simulink model "Messages4_2018a"  (R2018a)
settings: Solver=VariableStepAuto  StartTime=0.0  StopTime=0.2  RelTol=1e-3
settings Model: Creator=86188  LastModifiedBy=86188

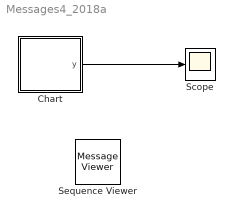
== system Messages4_2018a ==
  Chart : Stateflow chart  TreatAsAtomicUnit=on
  Scope : Scope
  Sequence Viewer : MessageViewer
  wires:
  Chart/1(y) -> Scope/1

== stateflow chart Messages4_2018a/Chart ==
  settings: updateMethod=DISCRETE  sampleTime=0.1
  state A
    en:
    f("en_A");
    M.data=3;
    send(M);
  state B
    en:
    f("en_B");
    y=1;
  state C
    en:
    f("en_C");
    y=2;
  state D
    en:
    f("en_D");
    y=3;
  (default) -> A
  A -> B : M[M.data==3]
  B -> C : [M.data==3]
  C -> D : [M.data==4]
  data: s function_input; M local; y output
  function f(s):
    | function f(s)
    |   fprintf(s+"\n");
